simulink model "CAN_TX"  (R2023b)
settings: Solver=FixedStepAuto  StartTime=0.0  StopTime=inf  FixedStep=0.01  RelTol=1e-3  EnableMultiTasking=on
libraries: stm32blockslib x2
settings Model: STM32="{\"CANWrite\":[{\"ID\":\"Exp06_Sim_CAN_TX:6\"},{\"ID\":\"Exp06_Sim_CAN_TX:1\"}]}"  Creator=dell  LastModifiedBy=dell
settings OptimizationCC: EnhancedBackFolding=on  PassReuseOutputArgsAs=Individual arguments  ZeroExternalMemoryAtStartup=off  ZeroInternalMemoryAtStartup=off  MaxStackSize=64  OptimizeBlockOrder=speed  DifferentSizesBufferReuse=on  OptimizationCustomize=off  EfficientTunableParamExpr=on
settings DebuggingCC: ParameterTunabilityLossMsg=error
settings HardwareCC: ProdBitPerPointer=32  ProdBitPerSizeT=32  ProdBitPerPtrDiffT=32  ProdLargestAtomicInteger=Long  ProdLargestAtomicFloat=Double  ProdWordSize=32  ProdLongLongMode=on  ProdHWDeviceType=ARM Compatible->ARM Cortex
settings SFSimCC: MATLABDynamicMemAlloc=off
settings RTWCC: Description=Embedded Coder  SystemTargetFile=ert.tlc  HardwareBoard=STM32F4xx Based  TemplateMakefile=ert_default_tmf  Toolchain=GNU Tools for ARM Embedded Processors
settings CodeAppCC: ForceParamTrailComments=on  IgnoreCustomStorageClasses=off  OperatorAnnotations=on  SimulinkDataObjDesc=on  SFDataObjDesc=on  InsertBlockDesc=on
settings ERTTargetCC: CodeReplacementLibrary=ARM Cortex-M  ExtModeTransport=2  ExtModeStaticAlloc=on  ExtModeStaticAllocSize=2048  ExtModeMexFile=ext_xcp  ExtModeIntrfLevel=Level2 - Open

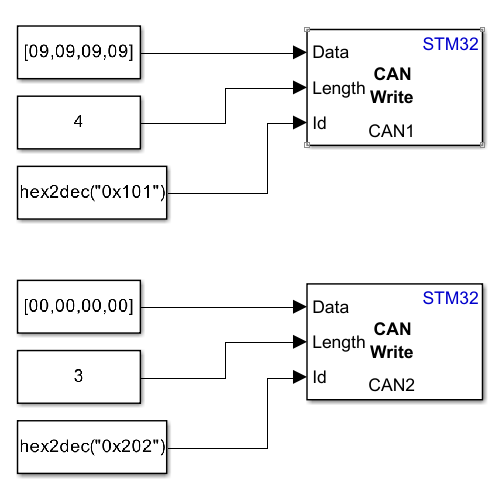
[thumbnail: Simulink's stored preview of the top-level diagram]
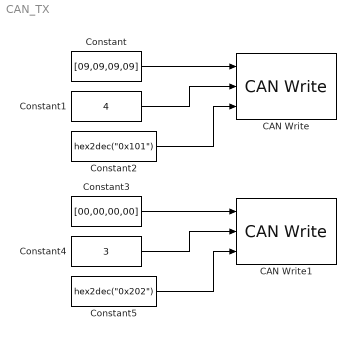
== system CAN_TX ==
  CAN Write : stm32blockslib/CAN Write  CANModule=CAN1  BlockMode=Transmit  OperationReadMode=Data  OperationWriteMode=Data  OutputTypeReadMode=Unpacked  DataFormatWriteMode=Raw data  ReadSource=FIFO 0  IdentifierTypeVia=Dialog  IdentifierType=Standard (11-bit identifier)  IdentifierVia=Inport  Identifier=100  DataLengthVia=Inport  DataLength=8  OutputIdType=off  TransmitRemoteFrame=off  OutputRemoteFrame=off  OutputTxFifoLevel=off  OutputRxFifoLevel=off  OutputStatus=off  Timeout=0.001  SampleTime=-1
      settings: LibrarySourceBlock=stm32f4xxblockslib/CAN Write
  CAN Write1 : stm32blockslib/CAN Write  CANModule=CAN2  BlockMode=Transmit  OperationReadMode=Data  OperationWriteMode=Data  OutputTypeReadMode=Unpacked  DataFormatWriteMode=Raw data  ReadSource=FIFO 0  IdentifierTypeVia=Dialog  IdentifierType=Standard (11-bit identifier)  IdentifierVia=Inport  Identifier=100  DataLengthVia=Inport  DataLength=8  OutputIdType=off  TransmitRemoteFrame=off  OutputRemoteFrame=off  OutputTxFifoLevel=off  OutputRxFifoLevel=off  OutputStatus=off  Timeout=0.001  SampleTime=-1
      settings: LibrarySourceBlock=stm32f4xxblockslib/CAN Write
  Constant : Constant  Value=[09,09,09,09]  OutDataTypeStr=uint8
  Constant1 : Constant  Value=4  OutDataTypeStr=uint8
  Constant2 : Constant  Value="hex2dec(\"0x101\")"
  Constant3 : Constant  Value=[00,00,00,00]  OutDataTypeStr=uint8
  Constant4 : Constant  Value=3  OutDataTypeStr=uint8
  Constant5 : Constant  Value="hex2dec(\"0x202\")"
  wires:
  Constant/1 -> CAN Write/1
  Constant1/1 -> CAN Write/2
  Constant2/1 -> CAN Write/3
  Constant4/1 -> CAN Write1/2
  Constant5/1 -> CAN Write1/3
  Constant3/1 -> CAN Write1/1
